simulink model "Engines"  (Simulink 8.2)
settings: Solver=ode45  StartTime=0.0  StopTime=10.0  RelTol=1e-3
undefined symbols (not defined in the file): MSSN
settings Model: Creator=Zach  LastModifiedBy=ASELab1

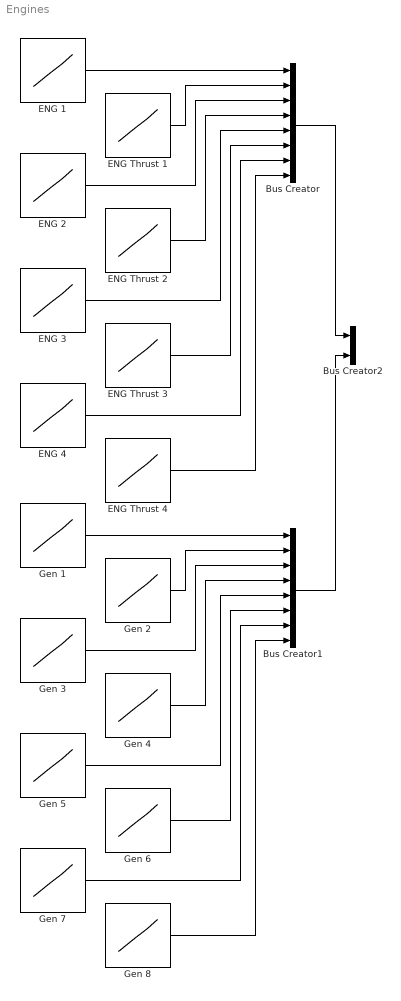
== system Engines ==
  Bus Creator : BusCreator  Inputs=8
  Bus Creator1 : BusCreator  Inputs=8
  Bus Creator2 : BusCreator  Inputs=2
  ENG 1 : Lookup  InputValues=MSSN.eng.time  Table=MSSN.eng.Eng1  LookUpMeth=Use Input Below
  ENG 2 : Lookup  InputValues=MSSN.eng.time  Table=MSSN.eng.Eng2  LookUpMeth=Use Input Below
  ENG 3 : Lookup  InputValues=MSSN.eng.time  Table=MSSN.eng.Eng3  LookUpMeth=Use Input Below
  ENG 4 : Lookup  InputValues=MSSN.eng.time  Table=MSSN.eng.Eng4  LookUpMeth=Use Input Below
  ENG Thrust 1 : Lookup  InputValues=MSSN.eng.time  Table=MSSN.eng.EngThrust1  LookUpMeth=Use Input Below
  ENG Thrust 2 : Lookup  InputValues=MSSN.eng.time  Table=MSSN.eng.EngThrust2  LookUpMeth=Use Input Below
  ENG Thrust 3 : Lookup  InputValues=MSSN.eng.time  Table=MSSN.eng.EngThrust3  LookUpMeth=Use Input Below
  ENG Thrust 4 : Lookup  InputValues=MSSN.eng.time  Table=MSSN.eng.EngThrust4  LookUpMeth=Use Input Below
  Gen 1 : Lookup  InputValues=MSSN.eng.time  Table=MSSN.eng.Gen1  LookUpMeth=Use Input Below
  Gen 2 : Lookup  InputValues=MSSN.eng.time  Table=MSSN.eng.Gen2  LookUpMeth=Use Input Below
  Gen 3 : Lookup  InputValues=MSSN.eng.time  Table=MSSN.eng.Gen3  LookUpMeth=Use Input Below
  Gen 4 : Lookup  InputValues=MSSN.eng.time  Table=MSSN.eng.Gen4  LookUpMeth=Use Input Below
  Gen 5 : Lookup  InputValues=MSSN.eng.time  Table=MSSN.eng.Gen5  LookUpMeth=Use Input Below
  Gen 6 : Lookup  InputValues=MSSN.eng.time  Table=MSSN.eng.Gen6  LookUpMeth=Use Input Below
  Gen 7 : Lookup  InputValues=MSSN.eng.time  Table=MSSN.eng.Gen7  LookUpMeth=Use Input Below
  Gen 8 : Lookup  InputValues=MSSN.eng.time  Table=MSSN.eng.Gen8  LookUpMeth=Use Input Below
  wires:
  ENG 1/1 -> Bus Creator/1
  ENG Thrust 1/1 -> Bus Creator/2
  ENG 2/1 -> Bus Creator/3
  ENG Thrust 2/1 -> Bus Creator/4
  ENG 3/1 -> Bus Creator/5
  ENG Thrust 3/1 -> Bus Creator/6
  ENG 4/1 -> Bus Creator/7
  ENG Thrust 4/1 -> Bus Creator/8
  Gen 1/1 -> Bus Creator1/1
  Gen 2/1 -> Bus Creator1/2
  Gen 3/1 -> Bus Creator1/3
  Gen 4/1 -> Bus Creator1/4
  Gen 5/1 -> Bus Creator1/5
  Gen 6/1 -> Bus Creator1/6
  Gen 7/1 -> Bus Creator1/7
  Gen 8/1 -> Bus Creator1/8
  Bus Creator/1 -> Bus Creator2/1
  Bus Creator1/1 -> Bus Creator2/2
